simulink model "Clutch_LockUp_Model"  (R2020a)
settings: Solver=VariableStepAuto  StartTime=0.0  StopTime=10.0  RelTol=1e-3
undefined symbols (not defined in the file): be, bv, le, lv
settings Model: Creator=NIKITA  LastModifiedBy=NIKITA

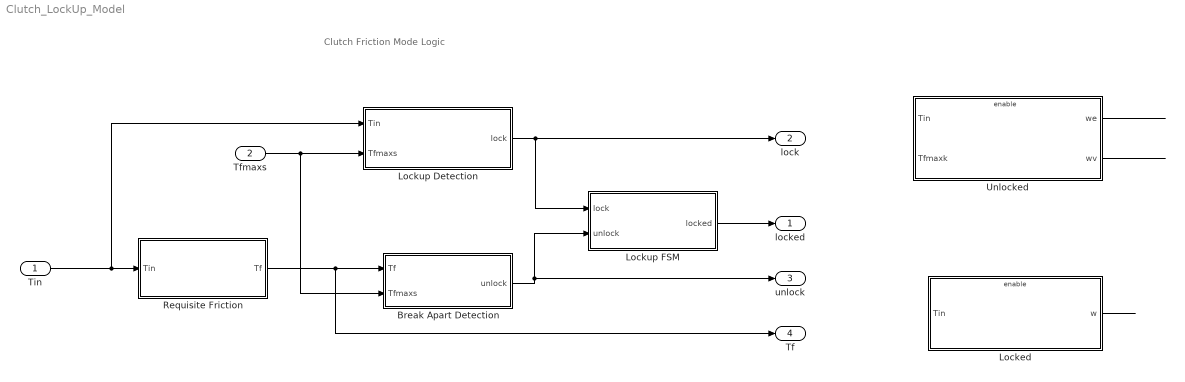
== system Clutch_LockUp_Model ==
  note: Clutch Friction Mode Logic
  Tin : Inport
  Tfmaxs : Inport  Port=2
  Break Apart Detection : Subsystem
  Locked : Subsystem
  Lockup Detection : Subsystem
  Lockup FSM : Subsystem
  Requisite Friction : Subsystem
  "Unlocked " : Subsystem
  locked : Outport
  lock : Outport  Port=2
  unlock : Outport  Port=3
  Tf : Outport  Port=4
  wires:
  ? -> "Unlocked "/1("Tin ")
  ? -> "Unlocked "/2(Tfmaxk)
  "Unlocked "/1(we) -> ?
  "Unlocked "/2(wv) -> ?
  ? -> Locked/1(Tin)
  Locked/1(w) -> ?
  Tin/1 -> Lockup Detection/1(Tin), Requisite Friction/1(Tin)
  Lockup Detection/1(lock) -> lock/1, Lockup FSM/1(lock)
  Break Apart Detection/1(unlock) -> unlock/1, Lockup FSM/2(unlock)
  Lockup FSM/1(locked) -> locked/1
  Requisite Friction/1(Tf) -> Tf/1, Break Apart Detection/1(Tf)
  Tfmaxs/1 -> Break Apart Detection/2(Tfmaxs), Lockup Detection/2(Tfmaxs)

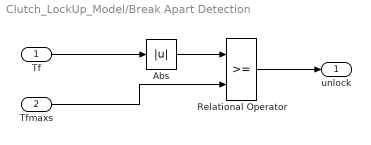
== system Clutch_LockUp_Model/Break Apart Detection ==
  Tf : Inport
  Tfmaxs : Inport  Port=2
  Abs : Abs
  Relational Operator : RelationalOperator  OutDataTypeStr=boolean  RndMeth=Simplest
  unlock : Outport
  wires:
  Abs/1 -> Relational Operator/1
  Tf/1 -> Abs/1
  Relational Operator/1 -> unlock/1
  Tfmaxs/1 -> Relational Operator/2

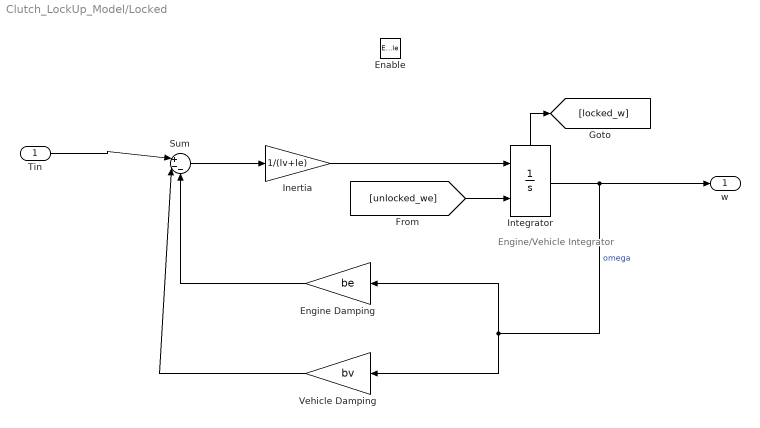
== system Clutch_LockUp_Model/Locked ==
  note: Engine/Vehicle
      | Integrator
  Tin : Inport
  Enable : EnablePort
  Engine Damping : Gain  Gain=be
  Inertia : Gain  Gain=1/(lv+le)
  Integrator : Integrator  InitialConditionSource=external  ShowStatePort=on
  Sum : Sum  Inputs=|+--
  Vehicle Damping : Gain  Gain=bv
  w : Outport
  wires:
  Inertia/1 -> Integrator/1
  Sum/1 -> Inertia/1
  Engine Damping/1 -> Sum/3
  Integrator/1 -> w/1, Engine Damping/1, Vehicle Damping/1  "omega"
  Vehicle Damping/1 -> Sum/2
  Integrator/State -> [locked_w]
  [unlocked_we] -> Integrator/2
  Tin/1 -> Sum/1

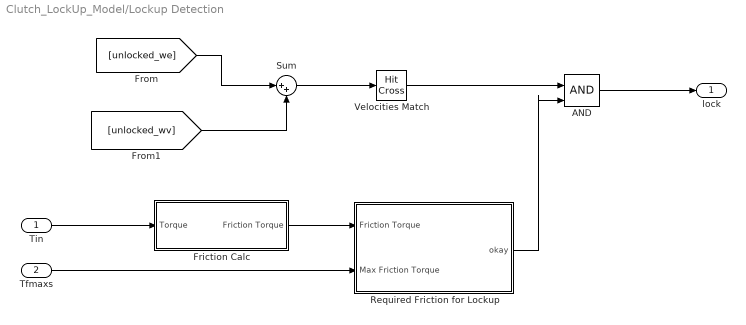
== system Clutch_LockUp_Model/Lockup Detection ==
  Tin : Inport
  Tfmaxs : Inport  Port=2
  "AND " : Logic  IconShape=distinctive  AllPortsSameDT=off  OutDataTypeStr=boolean
  Friction Calc : Subsystem
  Required Friction for Lockup : Subsystem
  Sum : Sum  Inputs=|++
  Velocities Match : HitCross
  lock : Outport
  wires:
  Friction Calc/1(Friction Torque) -> Required Friction for Lockup/1(Friction Torque)
  Tfmaxs/1 -> Required Friction for Lockup/2(Max Friction Torque)
  [unlocked_wv] -> Sum/2
  Sum/1 -> Velocities Match/1
  Tin/1 -> Friction Calc/1(Torque)
  "AND "/1 -> lock/1
  [unlocked_we] -> Sum/1
  Required Friction for Lockup/1(okay) -> "AND "/2
  Velocities Match/1 -> "AND "/1

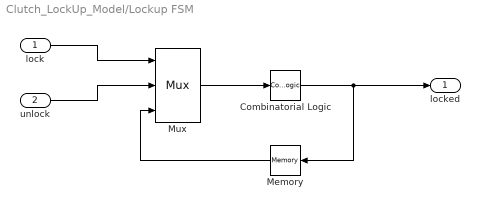
== system Clutch_LockUp_Model/Lockup FSM ==
  lock : Inport
  unlock : Inport  Port=2
  "Combinatorial Logic " : CombinatorialLogic
  "Memory " : Memory
  Mux : Mux  Inputs=3
  locked : Outport
  wires:
  "Combinatorial Logic "/1 -> locked/1, "Memory "/1
  unlock/1 -> Mux/2
  Mux/1 -> "Combinatorial Logic "/1
  "Memory "/1 -> Mux/3
  lock/1 -> Mux/1

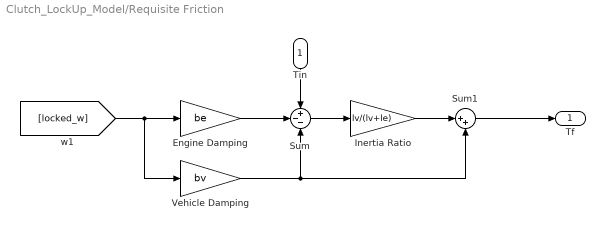
== system Clutch_LockUp_Model/Requisite Friction ==
  Tin : Inport
  Engine Damping : Gain  Gain=be
  Inertia Ratio : Gain  Gain=lv/(lv+le)
  Sum : Sum  Inputs=+--
  Sum1 : Sum  Inputs=|++
  Vehicle Damping : Gain  Gain=bv
  Tf : Outport
  wires:
  Tin/1 -> Sum/1
  Vehicle Damping/1 -> Sum1/2, Sum/3
  [locked_w] -> Vehicle Damping/1, Engine Damping/1
  Engine Damping/1 -> Sum/2
  Inertia Ratio/1 -> Sum1/1
  Sum1/1 -> Tf/1
  Sum/1 -> Inertia Ratio/1

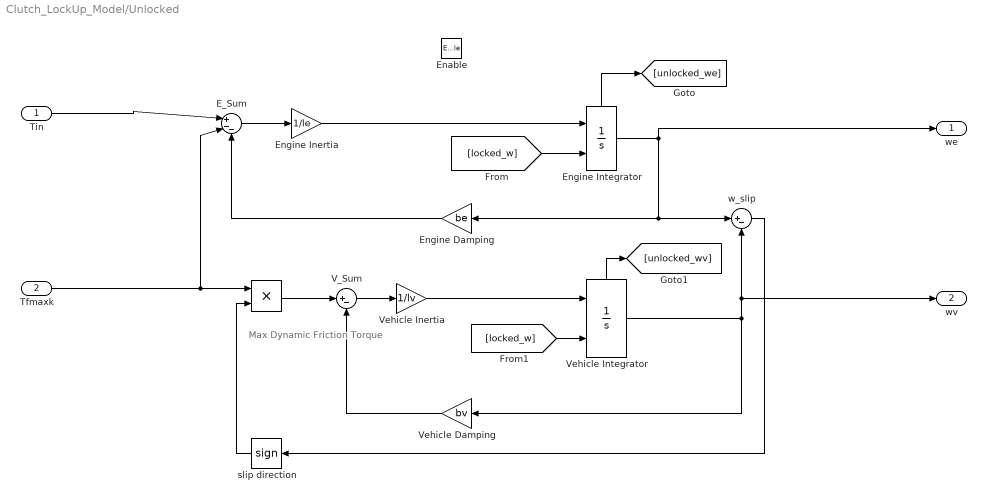
== system Clutch_LockUp_Model/Unlocked  ==
  note: Max
      | Dynamic
      | Friction
      | Torque
  "Tin " : Inport
  Tfmaxk : Inport  Port=2
  "Enable " : EnablePort  StatesWhenEnabling=reset
  " " : Product
  " Engine Integrator" : Integrator  InitialConditionSource=external  ShowStatePort=on
  E_Sum : Sum  Inputs=|+--
  Engine Damping : Gain  Gain=be
  Engine Inertia : Gain  Gain=1/le
  V_Sum : Sum  Inputs=|+-
  Vehicle Damping : Gain  Gain=bv
  Vehicle Inertia : Gain  Gain=1/lv
  Vehicle Integrator : Integrator  InitialConditionSource=external  ShowStatePort=on
  slip direction : Signum
  w_slip : Sum  Inputs=|+-
  we : Outport
  wv : Outport  Port=2
  wires:
  E_Sum/1 -> Engine Inertia/1
  slip direction/1 -> " "/2
  Vehicle Integrator/1 -> wv/1, w_slip/2, Vehicle Damping/1
  Tfmaxk/1 -> " "/1, E_Sum/2
  Engine Inertia/1 -> " Engine Integrator"/1
  " Engine Integrator"/1 -> we/1, w_slip/1, Engine Damping/1
  V_Sum/1 -> Vehicle Inertia/1
  w_slip/1 -> slip direction/1
  [locked_w] -> Vehicle Integrator/2
  " "/1 -> V_Sum/1
  Vehicle Inertia/1 -> Vehicle Integrator/1
  " Engine Integrator"/State -> [unlocked_we]
  [locked_w] -> " Engine Integrator"/2
  Vehicle Damping/1 -> V_Sum/2
  Engine Damping/1 -> E_Sum/3
  Vehicle Integrator/State -> [unlocked_wv]
  "Tin "/1 -> E_Sum/1

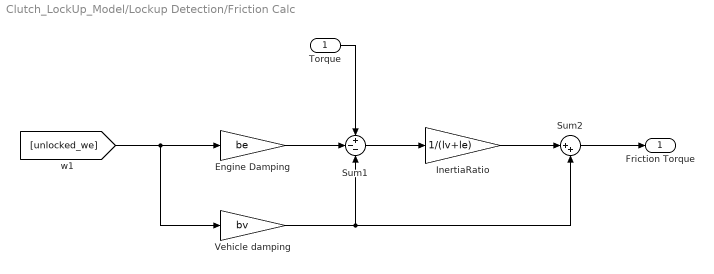
== system Clutch_LockUp_Model/Lockup Detection/Friction Calc ==
  Torque : Inport
  Engine Damping : Gain  Gain=be
  InertiaRatio : Gain  Gain=1/(lv+le)
  Sum1 : Sum  Inputs=+--
  Sum2 : Sum  Inputs=|++
  Vehicle damping : Gain  Gain=bv
  Friction Torque : Outport
  wires:
  Vehicle damping/1 -> Sum1/3, Sum2/2
  Engine Damping/1 -> Sum1/2
  InertiaRatio/1 -> Sum2/1
  Sum1/1 -> InertiaRatio/1
  Sum2/1 -> Friction Torque/1
  [unlocked_we] -> Vehicle damping/1, Engine Damping/1
  Torque/1 -> Sum1/1

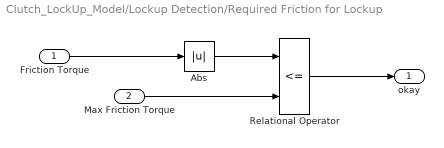
== system Clutch_LockUp_Model/Lockup Detection/Required Friction for Lockup ==
  Friction Torque : Inport
  Max Friction Torque : Inport  Port=2
  Abs : Abs
  Relational Operator : RelationalOperator  Operator=<=  OutDataTypeStr=boolean  RndMeth=Simplest
  okay : Outport
  wires:
  Abs/1 -> Relational Operator/1
  Relational Operator/1 -> okay/1
  Max Friction Torque/1 -> Relational Operator/2
  Friction Torque/1 -> Abs/1
